simulink model "godiva_R2019a"  (Simulink 9.3)
settings: Solver=FixedStepDiscrete  StartTime=0.0  StopTime=inf  RelTol=1e-3  EnableMultiTasking=on
InitFcn:
  | godiva_initfcn
StopFcn:
  | godiva_stopfcn
libraries: simulink x7
settings Model: Creator=alfnie  LastModifiedBy=alfnie
settings DataIOCC: LimitDataPoints=on
settings OptimizationCC: ExpressionDepthLimit=2147483647
settings DebuggingCC: SolverPrmCheckMsg=warning  StateNameClashWarn=warning
settings ConfigComp: CovExternalEMLEnable=on

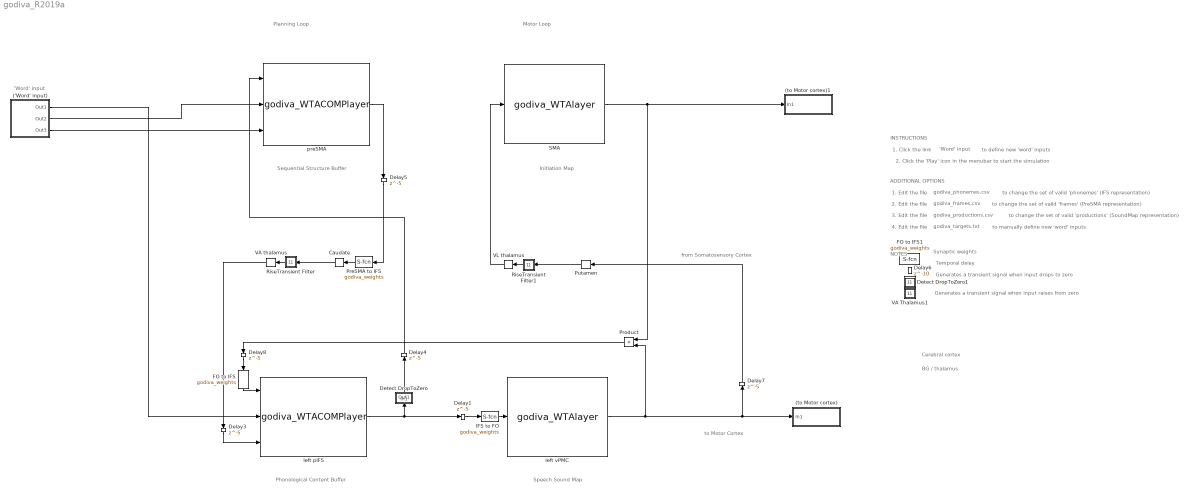
== system godiva_R2019a ==
  note: Cerebral cortex
  note: BG / thalamus
  note: godiva_phonemes.csv
  note: 1. Edit the file
  note: to change the set of valid 'phonemes' (IFS representation)
  note: godiva_frames.csv
  note: 2. Edit the file
  note: to change the set of valid 'frames' (PreSMA representation)
  note: godiva_productions.csv
  note: 3. Edit the file
  note: to change the set of valid 'productions' (SoundMap representation)
  note: ADDITIONAL OPTIONS
  note: to define new 'word' inputs
  note: 2. Click the 'Play' icon in the menubar to start the simulation
  note: INSTRUCTIONS
  note: Generates a transient signal when input drops to zero
  note: NOTES
  note: Generates a transient signal when input raises from zero
  note: Temporal delay
  note: Synaptic weights
  note: 'Word' input
  note: to Motor Cortex
  note: 'Word' input
  note: 1. Click the link
  note: godiva_targets.txt
  note: 4. Edit the file
  note: to manually define new 'word' inputs
  note: Sequential Structure Buffer
  note: Phonological Content Buffer
  note: Speech Sound Map
  note: Initiation Map
  note: Planning Loop
  note: Motor Loop
  note: from Somatosensory Cortex
  ('Word' input) : Subsystem
      mask Display:
      | port_label('output',1,'Phonemes')
      | port_label('output',2,'Frames')
      | port_label('output',3,'GO signal')
  (to Motor cortex) : Subsystem
      mask Display: port_label('input',1,'Motor Program')
  (to Motor cortex)1 : Subsystem
      mask Display: port_label('input',1,'GO signal')
  Caudate : Memory  InheritSampleTime=on  LinearizeAsDelay=on
  Delay{1,3..5,7..8} (6 alike) : Delay  DelayLength=5
  Delay6 : Delay  DelayLength=10
  Detect DropToZero : Subsystem
      mask Display: plot([0,.5,.5,1],[1,1,0,0])
  Detect DropToZero1 : Subsystem
      mask Display: plot([0,.5,.5,1],[1,1,0,0])
  FO to IFS : M-S-Function  FunctionName=godiva_weights  Parameters='godiva_weights_FO2IFS.mat'
      mask Display:
      | plot([0,.5,0.50,0.51,0.55,0.60,0.67,0.75,0.75,0.67,0.60,0.55,0.51,0.50],[.5,.5,0.50,0.35,0.21,0.10,0.02,0.00,1.00,0.98,0.90,0.79,0.65,0.50])
      | patch(.625+.8*([0.50,0.51,0.55,0.60,0.67,0.75,0.75,0.67,0.60,0.55,0.51,0.50]-.625),.5+.8*([0.50,0.35,0.21,0.10,0.02,0.00,1.00,0.98,0.90,0.79,0.65,0.50]-.5),1*[1,1,1])
  FO to IFS1 : M-S-Function  FunctionName=godiva_weights  Parameters='godiva_weights_PreSMA2IFS.mat'
      mask Display: plot([0,.5,0.50,0.51,0.55,0.60,0.67,0.75,0.75,0.67,0.60,0.55,0.51,0.50],[.5,.5,0.50,0.35,0.21,0.10,0.02,0.00,1.00,0.98,0.90,0.79,0.65,0.50])
  IFS to FO : M-S-Function  FunctionName=godiva_weights  Parameters='godiva_weights_IFS2FO.mat'
      mask Display:
      | plot([0,.5,0.50,0.51,0.55,0.60,0.67,0.75,0.75,0.67,0.60,0.55,0.51,0.50],[.5,.5,0.50,0.35,0.21,0.10,0.02,0.00,1.00,0.98,0.90,0.79,0.65,0.50])
      | patch(.625+.8*([0.50,0.51,0.55,0.60,0.67,0.75,0.75,0.67,0.60,0.55,0.51,0.50]-.625),.5+.8*([0.50,0.35,0.21,0.10,0.02,0.00,1.00,0.98,0.90,0.79,0.65,0.50]-.5),1*[1,1,1])
  PreSMA to IFS : M-S-Function  FunctionName=godiva_weights  Parameters='godiva_weights_PreSMA2IFS.mat'
      mask Display:
      | plot([0,.5,0.50,0.51,0.55,0.60,0.67,0.75,0.75,0.67,0.60,0.55,0.51,0.50],[.5,.5,0.50,0.35,0.21,0.10,0.02,0.00,1.00,0.98,0.90,0.79,0.65,0.50])
      | patch(.625+.8*([0.50,0.51,0.55,0.60,0.67,0.75,0.75,0.67,0.60,0.55,0.51,0.50]-.625),.5+.8*([0.50,0.35,0.21,0.10,0.02,0.00,1.00,0.98,0.90,0.79,0.65,0.50]-.5),1*[1,1,1])
  Product : Product
  Putamen : Memory  InheritSampleTime=on  LinearizeAsDelay=on
  RiseTransient Filter : Subsystem
      mask Display: plot([0,.5,.5,1],[0,0,1,1])
  RiseTransient Filter1 : Subsystem
      mask Display: plot([0,.5,.5,1],[0,0,1,1])
  SMA : M-S-Function  FunctionName=godiva_WTAlayer  Parameters='SMA',1, 0,1
      mask help: Plan / Choice competitive layer
      mask Display: image(imread('godiva_WTAlayer02.jpg'))
  VA Thalamus1 : Subsystem
      mask Display: plot([0,.5,.5,1],[0,0,1,1])
  VA thalamus : Memory  InheritSampleTime=on  LinearizeAsDelay=on
  VL thalamus : Memory  InheritSampleTime=on  LinearizeAsDelay=on
  left pIFS : M-S-Function  FunctionName=godiva_WTACOMPlayer  Parameters='IFS', 7 , 0, 1
      mask help: Plan / Choice competitive layer
      mask Display: image(imread('godiva_WTAlayer01.jpg'))
  left vPMC : M-S-Function  FunctionName=godiva_WTAlayer  Parameters='SSM',1, 0,1
      mask help: Plan / Choice competitive layer
      mask Display: image(imread('godiva_WTAlayer02.jpg'))
  preSMA : M-S-Function  FunctionName=godiva_WTACOMPlayer  Parameters='PreSMA', 1, 0, 1
      mask help: Plan / Choice competitive layer
      mask Display: image(imread('godiva_WTAlayer01.jpg'))
  wires:
  left pIFS/1 -> Detect DropToZero/1(In1), Delay1/1
  IFS to FO/1 -> left vPMC/1
  Delay1/1 -> IFS to FO/1
  Delay5/1 -> PreSMA to IFS/1
  RiseTransient Filter/1(Out1) -> VA thalamus/1
  Caudate/1 -> RiseTransient Filter/1(In1)
  PreSMA to IFS/1 -> Caudate/1
  VA thalamus/1 -> Delay3/1
  Delay3/1 -> left pIFS/3
  ('Word' input)/1(Out1) -> left pIFS/2
  FO to IFS/1 -> left pIFS/1
  ('Word' input)/2(Out2) -> preSMA/2
  ('Word' input)/3(Out3) -> preSMA/3
  Delay4/1 -> preSMA/1
  Detect DropToZero/1(Out1) -> Delay4/1
  Putamen/1 -> RiseTransient Filter1/1(In1)
  preSMA/1 -> Delay5/1
  Delay7/1 -> Putamen/1
  left vPMC/1 -> Product/2, (to Motor cortex)/1(In1), Delay7/1
  Delay8/1 -> FO to IFS/1
  RiseTransient Filter1/1(Out1) -> VL thalamus/1
  VL thalamus/1 -> SMA/1
  SMA/1 -> Product/1, (to Motor cortex)1/1(In1)
  Product/1 -> Delay8/1

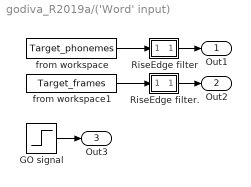
== system godiva_R2019a/('Word' input) ==
  GO signal : Step  Time=.010  SampleTime=.001
  RiseEdge filter : Subsystem
      mask Display: plot([0,.5,.5,1],[0,0,1,1])
  RiseEdge filter. : Subsystem
      mask Display: plot([0,.5,.5,1],[0,0,1,1])
  from workspace : FromWorkspace  VariableName=Target_phonemes  Interpolate=off  OutputAfterFinalValue=Holding final value
  from workspace1 : FromWorkspace  VariableName=Target_frames  Interpolate=off  OutputAfterFinalValue=Holding final value
  Out1 : Outport
  Out2 : Outport  Port=2
  Out3 : Outport  Port=3
  wires:
  from workspace/1 -> RiseEdge filter/1(In1)
  from workspace1/1 -> RiseEdge filter./1(In1)
  RiseEdge filter/1(Out1) -> Out1/1
  RiseEdge filter./1(Out1) -> Out2/1
  GO signal/1 -> Out3/1

== system godiva_R2019a/(to Motor cortex) ==
  In1 : Inport
  to workspace : ToWorkspace  VariableName=target_production  SampleTime=-1
  wires:
  In1/1 -> to workspace/1

== system godiva_R2019a/(to Motor cortex)1 ==
  In1 : Inport
  to workspace : ToWorkspace  VariableName=go_signal  SampleTime=-1
  wires:
  In1/1 -> to workspace/1

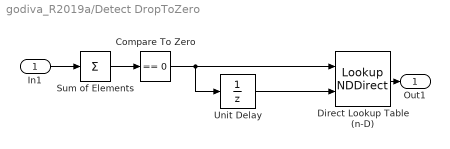
== system godiva_R2019a/Detect DropToZero ==
  In1 : Inport
  Compare To Zero : simulink/Logic and Bit Operations/Compare To Zero  relop===  OutDataTypeStr=boolean  ZeroCross=off
  Direct Lookup Table (n-D) : LookupNDDirect  Table=[0,0;1,0]
  Sum of Elements : Sum  Inputs=+
  Unit Delay : UnitDelay  InitialCondition=1  SampleTime=-1
  Out1 : Outport
  wires:
  Direct Lookup Table (n-D)/1 -> Out1/1
  Unit Delay/1 -> Direct Lookup Table (n-D)/2
  Compare To Zero/1 -> Direct Lookup Table (n-D)/1, Unit Delay/1
  In1/1 -> Sum of Elements/1
  Sum of Elements/1 -> Compare To Zero/1

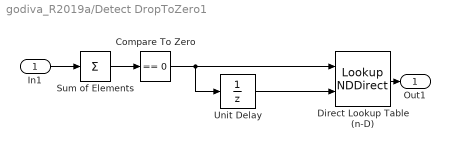
== system godiva_R2019a/Detect DropToZero1 ==
  In1 : Inport
  Compare To Zero : simulink/Logic and Bit Operations/Compare To Zero  relop===  OutDataTypeStr=boolean  ZeroCross=off
  Direct Lookup Table (n-D) : LookupNDDirect  Table=[0,0;1,0]
  Sum of Elements : Sum  Inputs=+
  Unit Delay : UnitDelay  InitialCondition=1  SampleTime=-1
  Out1 : Outport
  wires:
  Direct Lookup Table (n-D)/1 -> Out1/1
  Unit Delay/1 -> Direct Lookup Table (n-D)/2
  Compare To Zero/1 -> Direct Lookup Table (n-D)/1, Unit Delay/1
  In1/1 -> Sum of Elements/1
  Sum of Elements/1 -> Compare To Zero/1

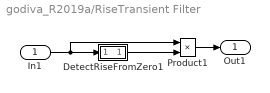
== system godiva_R2019a/RiseTransient Filter ==
  In1 : Inport
  DetectRiseFromZero1 : Subsystem
      mask Display: plot([0,.5,.5,1],[0,0,1,1])
  Product1 : Product  RndMeth=Zero
  Out1 : Outport
  wires:
  DetectRiseFromZero1/1(Out1) -> Product1/2
  In1/1 -> DetectRiseFromZero1/1(In1), Product1/1
  Product1/1 -> Out1/1

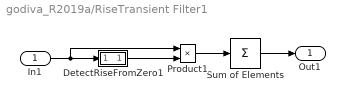
== system godiva_R2019a/RiseTransient Filter1 ==
  In1 : Inport
  DetectRiseFromZero1 : Subsystem
      mask Display: plot([0,.5,.5,1],[0,0,1,1])
  Product1 : Product  RndMeth=Zero
  Sum of Elements : Sum  Inputs=+
  Out1 : Outport
  wires:
  DetectRiseFromZero1/1(Out1) -> Product1/2
  In1/1 -> DetectRiseFromZero1/1(In1), Product1/1
  Product1/1 -> Sum of Elements/1
  Sum of Elements/1 -> Out1/1

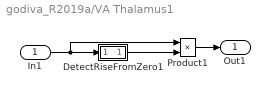
== system godiva_R2019a/VA Thalamus1 ==
  In1 : Inport
  DetectRiseFromZero1 : Subsystem
      mask Display: plot([0,.5,.5,1],[0,0,1,1])
  Product1 : Product  RndMeth=Zero
  Out1 : Outport
  wires:
  DetectRiseFromZero1/1(Out1) -> Product1/2
  In1/1 -> DetectRiseFromZero1/1(In1), Product1/1
  Product1/1 -> Out1/1

== system godiva_R2019a/('Word' input)/RiseEdge filter ==
  In1 : Inport
  DetectRiseFromZero1 : Subsystem
      mask Display: plot([0,.5,.5,1],[0,0,1,1])
  Product1 : Product  RndMeth=Zero
  Out1 : Outport
  wires:
  DetectRiseFromZero1/1(Out1) -> Product1/2
  In1/1 -> DetectRiseFromZero1/1(In1), Product1/1
  Product1/1 -> Out1/1

== system godiva_R2019a/('Word' input)/RiseEdge filter. ==
  In1 : Inport
  DetectRiseFromZero1 : Subsystem
      mask Display: plot([0,.5,.5,1],[0,0,1,1])
  Product1 : Product  RndMeth=Zero
  Out1 : Outport
  wires:
  DetectRiseFromZero1/1(Out1) -> Product1/2
  In1/1 -> DetectRiseFromZero1/1(In1), Product1/1
  Product1/1 -> Out1/1

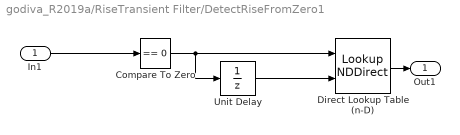
== system godiva_R2019a/RiseTransient Filter/DetectRiseFromZero1 ==
  In1 : Inport
  Compare To Zero : simulink/Logic and Bit Operations/Compare To Zero  relop===  OutDataTypeStr=boolean  ZeroCross=off
  Direct Lookup Table (n-D) : LookupNDDirect  Table=[0,1;0,0]
  Unit Delay : UnitDelay  InitialCondition=1  SampleTime=-1
  Out1 : Outport
  wires:
  Direct Lookup Table (n-D)/1 -> Out1/1
  Unit Delay/1 -> Direct Lookup Table (n-D)/2
  Compare To Zero/1 -> Direct Lookup Table (n-D)/1, Unit Delay/1
  In1/1 -> Compare To Zero/1

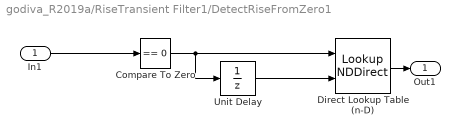
== system godiva_R2019a/RiseTransient Filter1/DetectRiseFromZero1 ==
  In1 : Inport
  Compare To Zero : simulink/Logic and Bit Operations/Compare To Zero  relop===  OutDataTypeStr=boolean  ZeroCross=off
  Direct Lookup Table (n-D) : LookupNDDirect  Table=[0,1;0,0]
  Unit Delay : UnitDelay  InitialCondition=1  SampleTime=-1
  Out1 : Outport
  wires:
  Direct Lookup Table (n-D)/1 -> Out1/1
  Unit Delay/1 -> Direct Lookup Table (n-D)/2
  Compare To Zero/1 -> Direct Lookup Table (n-D)/1, Unit Delay/1
  In1/1 -> Compare To Zero/1

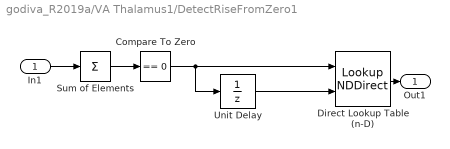
== system godiva_R2019a/VA Thalamus1/DetectRiseFromZero1 ==
  In1 : Inport
  Compare To Zero : simulink/Logic and Bit Operations/Compare To Zero  relop===  OutDataTypeStr=boolean  ZeroCross=off
  Direct Lookup Table (n-D) : LookupNDDirect  Table=[0,1;0,0]
  Sum of Elements : Sum  Inputs=+
  Unit Delay : UnitDelay  InitialCondition=1  SampleTime=-1
  Out1 : Outport
  wires:
  Direct Lookup Table (n-D)/1 -> Out1/1
  Unit Delay/1 -> Direct Lookup Table (n-D)/2
  Compare To Zero/1 -> Direct Lookup Table (n-D)/1, Unit Delay/1
  In1/1 -> Sum of Elements/1
  Sum of Elements/1 -> Compare To Zero/1

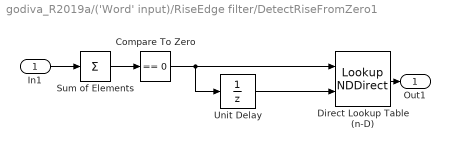
== system godiva_R2019a/('Word' input)/RiseEdge filter/DetectRiseFromZero1 ==
  In1 : Inport
  Compare To Zero : simulink/Logic and Bit Operations/Compare To Zero  relop===  OutDataTypeStr=boolean  ZeroCross=off
  Direct Lookup Table (n-D) : LookupNDDirect  Table=[0,1;0,0]
  Sum of Elements : Sum  Inputs=+
  Unit Delay : UnitDelay  InitialCondition=1  SampleTime=-1
  Out1 : Outport
  wires:
  Direct Lookup Table (n-D)/1 -> Out1/1
  Unit Delay/1 -> Direct Lookup Table (n-D)/2
  Compare To Zero/1 -> Direct Lookup Table (n-D)/1, Unit Delay/1
  In1/1 -> Sum of Elements/1
  Sum of Elements/1 -> Compare To Zero/1

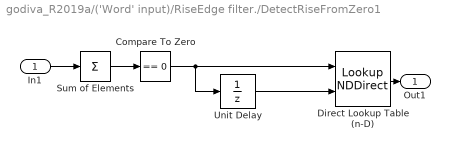
== system godiva_R2019a/('Word' input)/RiseEdge filter./DetectRiseFromZero1 ==
  In1 : Inport
  Compare To Zero : simulink/Logic and Bit Operations/Compare To Zero  relop===  OutDataTypeStr=boolean  ZeroCross=off
  Direct Lookup Table (n-D) : LookupNDDirect  Table=[0,1;0,0]
  Sum of Elements : Sum  Inputs=+
  Unit Delay : UnitDelay  InitialCondition=1  SampleTime=-1
  Out1 : Outport
  wires:
  Direct Lookup Table (n-D)/1 -> Out1/1
  Unit Delay/1 -> Direct Lookup Table (n-D)/2
  Compare To Zero/1 -> Direct Lookup Table (n-D)/1, Unit Delay/1
  In1/1 -> Sum of Elements/1
  Sum of Elements/1 -> Compare To Zero/1
